simulink model "DistrubanceRejection_withObserver"  (R2017b)
settings: Solver=ode4  StartTime=0.0  StopTime=50  FixedStep=0.05  RelTol=1e-3  EnableMultiTasking=on
undefined symbols (not defined in the file or in its folder): A, Aa, Aw, B, Ba, Bv, C, Ca, Cw, K1, K2, L, w0, x0, xhat0
settings Model: Creator=roga  LastModifiedBy=Roberto
settings DataIOCC: LimitDataPoints=on  SaveFormat=Array
settings OptimizationCC: LifeSpan=inf
settings DebuggingCC: UnderspecifiedInitializationDetection=Classic  MergeDetectMultiDrivingBlocksExec=none  SolverPrmCheckMsg=warning  SFUnexpectedBacktrackingDiag=warning  SFNoUnconditionalDefaultTransitionDiag=warning  SFExecutionAtInitializationDiag=none
settings HardwareCC: ProdBitPerPointer=32  ProdBitPerSizeT=32  ProdBitPerPtrDiffT=32  ProdLargestAtomicFloat=None  ProdIntDivRoundTo=Undefined  ProdEndianess=Unspecified  ProdWordSize=32  ProdHWDeviceType=32-bit Generic
settings ModelReferenceCC: PropagateSignalLabelsOutOfModel=off
settings CodeAppCC: StateflowObjectComments=on
settings GRTTargetCC: TargetLangStandard=C89/C90 (ANSI)  GeneratePreprocessorConditionals=Disable all
settings ConfigComp: CovMetricSettings=dw  CovHtmlReporting=on  CovSaveCumulativeToWorkspaceVar=on  CovSaveSingleToWorkspaceVar=on  CovExternalEMLEnable=off  CovSFcnEnable=off

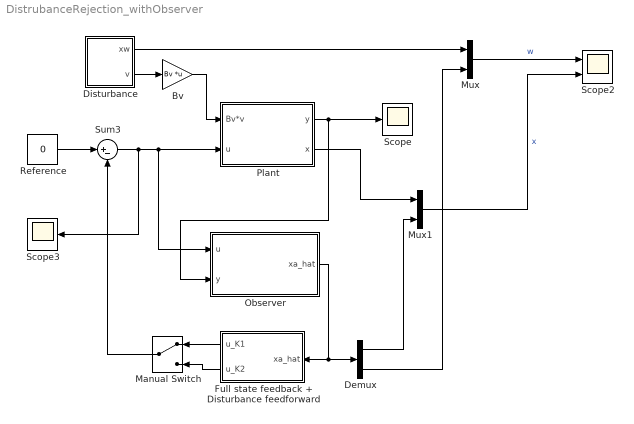
== system DistrubanceRejection_withObserver ==
  Bv : Gain  Gain=Bv  Multiplication=Matrix(K*u) (u vector)
  Demux : Demux  Outputs=2
  Disturbance : Subsystem
  Full state feedback + Disturbance feedforward : Subsystem
  Manual Switch : ManualSwitch
  Mux : Mux  Inputs=2
  Mux1 : Mux  Inputs=2
  Observer : Subsystem
  Plant : Subsystem
  Reference : Constant  Value=0
  Scope : Scope
  Scope2 : Scope  NumInputPorts=2
  Scope3 : Scope
  Sum3 : Sum  Inputs=|+-
  wires:
  Sum3/1 -> Scope3/1, Plant/2(u), Observer/1(u)
  Reference/1 -> Sum3/1
  Mux/1 -> Scope2/1  "w"
  Mux1/1 -> Scope2/2  "x"
  Demux/1 -> Mux1/2
  Observer/1(xa_hat) -> Demux/1, Full state feedback + Disturbance feedforward/1(xa_hat)
  Full state feedback + Disturbance feedforward/1(u_K1) -> Manual Switch/1
  Full state feedback + Disturbance feedforward/2(u_K2) -> Manual Switch/2
  Plant/1(y) -> Scope/1, Observer/2(y)
  Plant/2(x) -> Mux1/1
  Disturbance/2(v) -> Bv/1
  Disturbance/1(xw) -> Mux/1
  Demux/2 -> Mux/2
  Manual Switch/1 -> Sum3/2
  Bv/1 -> Plant/1(Bv*v)

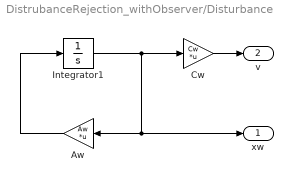
== system DistrubanceRejection_withObserver/Disturbance ==
  Aw : Gain  Gain=Aw  Multiplication=Matrix(K*u) (u vector)
  Cw : Gain  Gain=Cw  Multiplication=Matrix(K*u) (u vector)
  Integrator1 : Integrator  InitialCondition=w0
  xw : Outport
  v : Outport  Port=2
  wires:
  Aw/1 -> Integrator1/1
  Integrator1/1 -> Cw/1, xw/1, Aw/1
  Cw/1 -> v/1

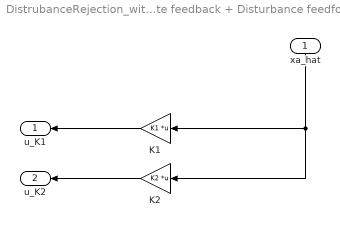
== system DistrubanceRejection_withObserver/Full state feedback + Disturbance feedforward ==
  xa_hat : Inport
  K1 : Gain  Gain=K1  Multiplication=Matrix(K*u) (u vector)
  K2 : Gain  Gain=K2  Multiplication=Matrix(K*u) (u vector)
  u_K1 : Outport
  u_K2 : Outport  Port=2
  wires:
  K1/1 -> u_K1/1
  K2/1 -> u_K2/1
  xa_hat/1 -> K2/1, K1/1

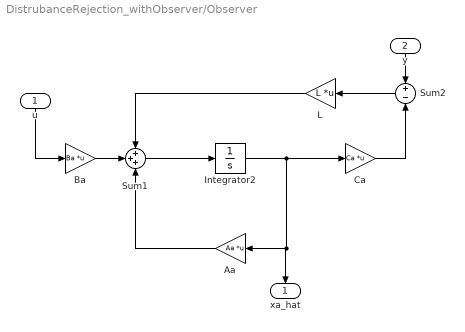
== system DistrubanceRejection_withObserver/Observer ==
  u : Inport
  y : Inport  Port=2
  Aa : Gain  Gain=Aa  Multiplication=Matrix(K*u) (u vector)
  Ba : Gain  Gain=Ba  Multiplication=Matrix(K*u) (u vector)
  Ca : Gain  Gain=Ca  Multiplication=Matrix(K*u) (u vector)
  Integrator2 : Integrator  InitialCondition=xhat0
  L : Gain  Gain=L  Multiplication=Matrix(K*u) (u vector)
  Sum1 : Sum  Inputs=+++
  Sum2 : Sum  Inputs=+-
  xa_hat : Outport
  wires:
  Ba/1 -> Sum1/2
  Sum1/1 -> Integrator2/1
  Aa/1 -> Sum1/3
  Ca/1 -> Sum2/2
  Sum2/1 -> L/1
  L/1 -> Sum1/1
  u/1 -> Ba/1
  Integrator2/1 -> Aa/1, xa_hat/1, Ca/1
  y/1 -> Sum2/1

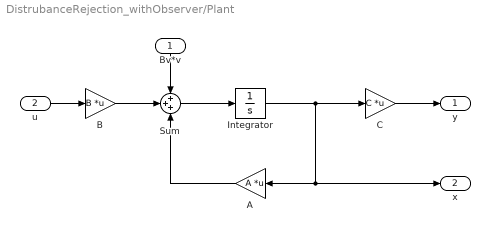
== system DistrubanceRejection_withObserver/Plant ==
  Bv*v : Inport
  u : Inport  Port=2
  A : Gain  Gain=A  Multiplication=Matrix(K*u) (u vector)
  B : Gain  Gain=B  Multiplication=Matrix(K*u) (u vector)
  C : Gain  Gain=C  Multiplication=Matrix(K*u) (u vector)
  Integrator : Integrator  InitialCondition=x0
  Sum : Sum  Inputs=+++
  y : Outport
  x : Outport  Port=2
  wires:
  Sum/1 -> Integrator/1
  A/1 -> Sum/3
  B/1 -> Sum/2
  Integrator/1 -> C/1, x/1, A/1
  C/1 -> y/1
  Bv*v/1 -> Sum/1
  u/1 -> B/1
